simulink model "PMSM"  (R2022a)
settings: Solver=ode23t  StartTime=0.0  StopTime=11  MaxStep=1e-6  RelTol=1e-3
values from neighbouring files (symbols this model uses):
  eps_startup = f/t_startup    (= 40.8333333333)    [PMSM.m]
  J = 0.00000600    (= 6e-06)    [PMSM.m]
  Ls = 0.0002700    (= 0.00027)    [PMSM.m]
  psi = 0.0043319    [PMSM.m]
  Rs = 0.600    (= 0.6)    [PMSM.m]
  t_startup = 10    [PMSM.m]
  zp = 7    [PMSM.m]
libraries: fl_lib x11, nesl_utility x10, ee_lib x1
settings Model: Creator=63250  LastModifiedBy=81502

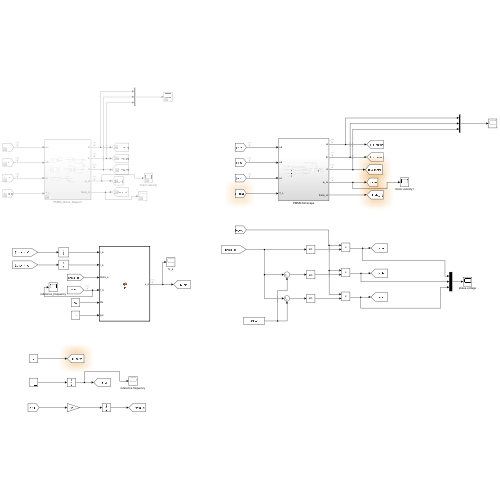
[thumbnail: Simulink's stored preview of the top-level diagram]
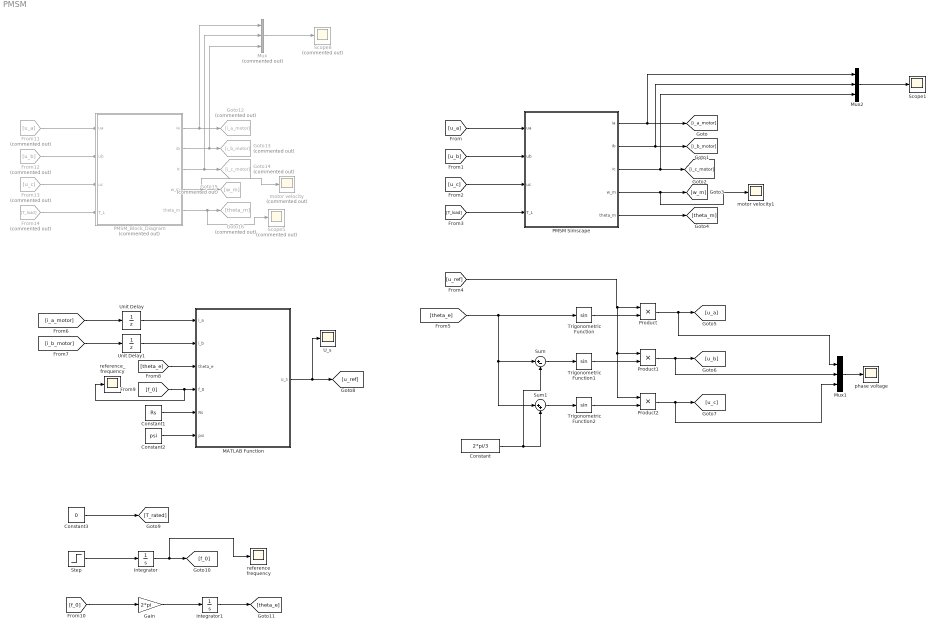
== system PMSM ==
  Constant : Constant  Value=2*pi/3
  Constant1 : Constant  Value=Rs
  Constant2 : Constant  Value=psi
  Constant3 : Constant  Value=0
  From11 : From  Commented=on  GotoTag=u_a
  From12 : From  Commented=on  GotoTag=u_b
  From13 : From  Commented=on  GotoTag=u_c
  From14 : From  Commented=on  GotoTag=T_load
  Gain : Gain  Gain=2*pi
  Goto12 : Goto  Commented=on  GotoTag=i_a_motor
  Goto13 : Goto  Commented=on  GotoTag=i_b_motor
  Goto14 : Goto  Commented=on  GotoTag=i_c_motor
  Goto15 : Goto  Commented=on  GotoTag=w_m
  Goto16 : Goto  Commented=on  GotoTag=theta_m
  Integrator : Integrator
  Integrator1 : Integrator
  MATLAB Function : MATLAB Function  TreatAsAtomicUnit=on
  Mux : Mux  Commented=on  Inputs=3
  Mux1 : Mux  Inputs=3
  Mux2 : Mux  Inputs=3
  PMSM Simscape : Subsystem
  PMSM_Block_Diagram : Subsystem  Commented=on
  Product : Product
  Product1 : Product
  Product2 : Product
  Scope1 : Scope
  Scope5 : Scope  Commented=on
  Scope8 : Scope  Commented=on
  Step : Step  Time=t_startup  Before=eps_startup  After=0  OutDataTypeStr=Inherit: Inherit via back propagation  SampleTime=0
  Sum : Sum  Inputs=|+-
  Sum1 : Sum  Inputs=|++
  Trigonometric Function : Trigonometry
  Trigonometric Function1 : Trigonometry
  Trigonometric Function2 : Trigonometry
  U_s : Scope
  Unit Delay : UnitDelay  SampleTime=-1  HasFrameUpgradeWarning=on
  Unit Delay1 : UnitDelay  SampleTime=-1  HasFrameUpgradeWarning=on
  motor velocity : Scope  Commented=on
  motor velocity1 : Scope
  phase voltage : Scope
  reference frequency : Scope
  reference_frequency : Scope
  wires:
  [u_a] -> PMSM Simscape/1(ua)
  [u_b] -> PMSM Simscape/2(ub)
  [u_c] -> PMSM Simscape/3(uc)
  [T_load] -> PMSM Simscape/4(T_L)
  PMSM Simscape/5(theta_m) -> [theta_m]
  PMSM Simscape/4(w_m) -> motor velocity1/1, [w_m]
  [theta_e] -> Sum/1, Sum1/1, Trigonometric Function/1
  Sum/1 -> Trigonometric Function1/1
  Sum1/1 -> Trigonometric Function2/1
  Constant/1 -> Sum1/2, Sum/2
  Trigonometric Function2/1 -> Product2/2
  Trigonometric Function1/1 -> Product1/2
  Trigonometric Function/1 -> Product/2
  [u_ref] -> Product2/1, Product1/1, Product/1
  [i_a_motor] -> Unit Delay/1
  [i_b_motor] -> Unit Delay1/1
  MATLAB Function/1(u_s) -> U_s/1, [u_ref]
  Unit Delay/1 -> MATLAB Function/1(i_a)
  Unit Delay1/1 -> MATLAB Function/2(i_b)
  [theta_e] -> MATLAB Function/3(theta_e)
  [f_0] -> reference_frequency/1, MATLAB Function/4(f_0)
  Constant1/1 -> MATLAB Function/5(Rs)
  Constant2/1 -> MATLAB Function/6(psi)
  Constant3/1 -> [T_rated]
  Integrator1/1 -> [theta_e]
  Integrator/1 -> reference frequency/1, [f_0]
  Step/1 -> Integrator/1
  [f_0] -> Gain/1
  Gain/1 -> Integrator1/1
  From11/1 -> PMSM_Block_Diagram/1(ua)
  From13/1 -> PMSM_Block_Diagram/3(uc)
  From14/1 -> PMSM_Block_Diagram/4(T_L)
  From12/1 -> PMSM_Block_Diagram/2(ub)
  PMSM_Block_Diagram/2(ib) -> Mux/3, Goto13/1
  PMSM_Block_Diagram/5(theta_m) -> Scope5/1, Goto16/1
  PMSM_Block_Diagram/4(w_m) -> motor velocity/1, Goto15/1
  Mux/1 -> Scope8/1
  PMSM_Block_Diagram/3(ic) -> Goto14/1, Mux/2
  PMSM_Block_Diagram/1(ia) -> Mux/1, Goto12/1
  Mux1/1 -> phase voltage/1
  Product2/1 -> Mux1/3, [u_c]
  Product/1 -> Mux1/1, [u_a]
  Product1/1 -> Mux1/2, [u_b]
  Mux2/1 -> Scope1/1
  PMSM Simscape/1(ia) -> Mux2/1, [i_a_motor]
  PMSM Simscape/3(ic) -> Mux2/3, [i_c_motor]
  PMSM Simscape/2(ib) -> Mux2/2, [i_b_motor]

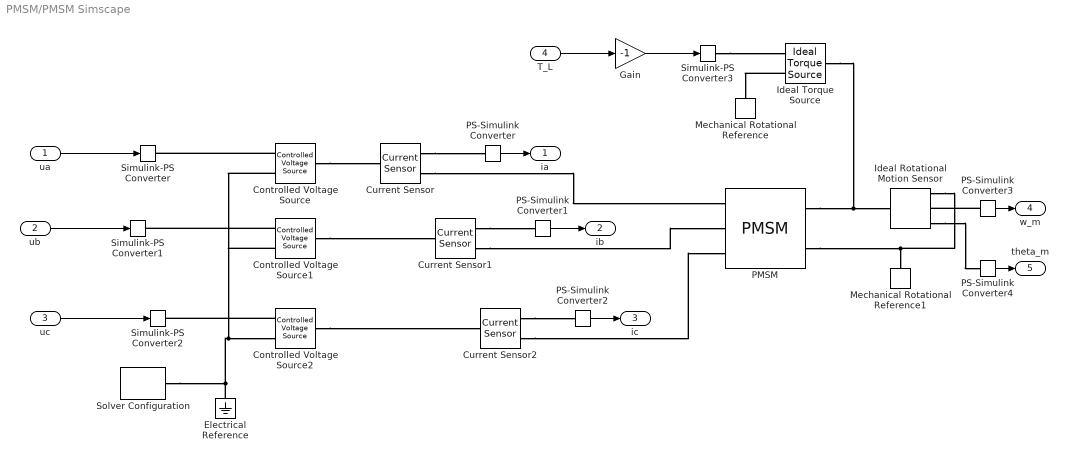
== system PMSM/PMSM Simscape ==
  ua : Inport
  ub : Inport  Port=2
  uc : Inport  Port=3
  T_L : Inport  Port=4
  Controlled Voltage Source : fl_lib/Electrical/Electrical Sources/Controlled Voltage Source
      settings: SourceProductBaseCode=PW,SS,VE
  Controlled Voltage Source1 : fl_lib/Electrical/Electrical Sources/Controlled Voltage Source
      settings: SourceProductBaseCode=PW,SS,VE
  Controlled Voltage Source2 : fl_lib/Electrical/Electrical Sources/Controlled Voltage Source
      settings: SourceProductBaseCode=PW,SS,VE
  Current Sensor : fl_lib/Electrical/Electrical Sensors/Current Sensor
      settings: SourceProductBaseCode=PW,SS,VE
  Current Sensor1 : fl_lib/Electrical/Electrical Sensors/Current Sensor
      settings: SourceProductBaseCode=PW,SS,VE
  Current Sensor2 : fl_lib/Electrical/Electrical Sensors/Current Sensor
      settings: SourceProductBaseCode=PW,SS,VE
  Electrical Reference : fl_lib/Electrical/Electrical Elements/Electrical Reference
      settings: SourceProductBaseCode=PW,SS,VE
  Gain : Gain  Gain=-1
  Ideal Rotational Motion Sensor : fl_lib/Mechanical/Mechanical Sensors/Ideal Rotational Motion Sensor  wrap_angle=simscape.enum.onoff.off  offset=0 rad
      settings: SourceProductBaseCode=PW,SS,VE
  Ideal Torque Source : fl_lib/Mechanical/Mechanical Sources/Ideal Torque Source
      settings: SourceProductBaseCode=PW,SS,VE
  Mechanical Rotational Reference : fl_lib/Mechanical/Rotational Elements/Mechanical Rotational Reference
      settings: SourceProductBaseCode=PW,SS,VE
  Mechanical Rotational Reference1 : fl_lib/Mechanical/Rotational Elements/Mechanical Rotational Reference
      settings: SourceProductBaseCode=PW,SS,VE
  PMSM : ee_lib/Electromechanical/Permanent Magnet/PMSM  port_option=ee.enum.threePhasePort.expanded  winding_type=ee.enum.statorconnection.wye  machine_param=ee.enum.pmsm.parameterization.constant  nPolePairs=zp  pmflux_param=ee.enum.pmflux.fluxlinkage  pm_flux_linkage=psi Wb  torque_constant=0.18 N*m/A  back_emf_constant=0.18 V*s/rad  stator_param=ee.enum.statorparam.LdLqL0  Ld=Ls H  Lq=Ls H  idVec=[-200, 0, 200] A  iqVec=[-200, 0, 200] A  LdMatrix=0.0002 * ones(3, 3) H  LqMatrix=0.0002 * ones(3, 3) H  PmMatrix=0.1 * ones(3, 3) Wb  ktMatrix=0.18 * ones(3, 3) N*m/A  keMatrix=0.18 * ones(3, 3) V*s/rad  L0=Rs H  Ls=0.0002 H  Lm=-0.00002 H  Ms=0.00002 H  Rs=Rs Ohm  zero_sequence=ee.enum.park.zerosequence.exclude  axes_param=ee.enum.rotorangle.daxis  loss_param=ee.enum.ironloss.none  losses_oc=[0, 0, 0] W  losses_sc=[0, 0, 0] W  f_losses=60 Hz  Isc_losses=95 A  J=J kg*m^2  lam=0 N*m*s/rad  i_d_specify=off  i_d_priority=None  i_d=0 A  i_d_nominal_specify=off  i_d_nominal_unit=A  i_d_nominal_value=1  i_q_specify=off  i_q_priority=None  i_q=0 A  i_q_nominal_specify=off  i_q_nominal_unit=A  i_q_nominal_value=1  torque_specify=off  torque_priority=None  torque=0 N*m  torque_nominal_specify=off  torque_nominal_unit=N*m  torque_nominal_value=1  angular_velocity_specify=off  angular_velocity_priority=High  angular_velocity=0 rpm  angular_velocity_nominal_specify=off  angular_velocity_nominal_unit=rpm  angular_velocity_nominal_value=1  angular_position_specify=off  angular_position_priority=High  angular_position=0 deg  angular_position_nominal_specify=off  angular_position_nominal_unit=deg  angular_position_nominal_value=1  alpha=3.93e-3 1/K  alpha_flux=-0.001 1/K  Tmeas=298.15 K  stator_thermal_mass=100 J/K  rotor_thermal_mass=200 J/K  Rm_percent_rotor=90  Rd_percent_rotor=30  temperatureA_specify=off  temperatureA_priority=High  temperatureA=25 degC  temperatureA_nominal_specify=off  temperatureA_nominal_unit=degC  temperatureA_nominal_value=1  temperatureB_specify=off  temperatureB_priority=High  temperatureB=25 degC  temperatureB_nominal_specify=off  temperatureB_nominal_unit=degC  temperatureB_nominal_value=1  temperatureC_specify=off  temperatureC_priority=High  temperatureC=25 degC  temperatureC_nominal_specify=off  temperatureC_nominal_unit=degC  temperatureC_nominal_value=1  temperatureR_specify=off  temperatureR_priority=High  temperatureR=25 degC  temperatureR_nominal_specify=off  temperatureR_nominal_unit=degC  temperatureR_nominal_value=1
      settings: InternalSimscapePortConfiguration="{\"Bottom\":[],\"Left\":[{\"id\":\"a\",\"label\":\"a\",\"type\":\"foundation.electrical.electrical\"},{\"id\":\"b\",\"label\":\"b\",\"type\":\"foundation.electrical.electrical\"},{\"id\":\"c\",\"label\":\"c\",\"type\":\"foundation.electrical.electrical\"}],\"Right\":[{\"id\":\"R\",\"label\":\"R\",\"type\":\"foundation.mechanical.rotational.rotational\"},{\"id\":\"C\",\"label\":\"C\",\"type\":\"foundation.mechanical.rotational.rotational\"}],\"Top\":[]}"
  PS-Simulink Converter{,1..4} (5 alike) : nesl_utility/PS-Simulink Converter  PhysicalDomain=network_engine_domain  SubClassName=ps_output  LeftPortType=input  RightPortType=output  PseudoPeriodic=off  Frequencies=[]  VectorFormat=inherit  Unit=inherit  AffineConversion=off
      settings: SourceProductBaseCode=SS,PW,VE
  Simulink-PS Converter{,1..3} (4 alike) : nesl_utility/Simulink-PS Converter  PhysicalDomain=network_engine_domain  SubClassName=ps_input  LeftPortType=input  RightPortType=output  PseudoPeriodic=off  Frequencies=[]  NoiseDistribution=none  NoiseParameters=[]  Unit=1  AffineConversion=off  FilteringAndDerivatives=provide  SimscapeFilterOrder=1  InputFilterTimeConstant=0.001  UdotUserProvided=0
      settings: SourceProductBaseCode=SS,PW,VE
  Solver Configuration : nesl_utility/Solver Configuration  PhysicalDomain=network_engine_domain  SubClassName=solver  LeftPortType=input  RightPortType=generic  Tones=[]  Harmonics=[]  SimulateNoise=off  Profile=off  UseLocalSampling=off  EnableSwitchedLinearOptims=on  FrequencyDomain=off  UseCCode=off  RelTol=0.001  AbsTol=0.001  MinStep=1e-09  ToWorkspace=off  RevertToSquareIcSolve=off  NumHomotopyIterations=100  PhasorMode=off  PhasorModeNumHarmonics=1  IndexReductionMethod=DerivativeReplacement  DoDC=off  ResidualTolerance=1e-09  UseLocalSolver=off  LocalSolverChoice=NE_BACKWARD_EULER_ADVANCER  LocalSolverSampleTime=0.001  DoFixedCost=off  MaxNonlinIter=3  MaxModeIter=2  ComputeImpulses=off  ImpulseIterations=2  LinearAlgebra=auto  LinearAlgebraNumThread=0  EquationFormulation=NE_TIME_EF  DelaysMemoryBudget=1024  AutomaticFiltering=on  FilteringTimeConstant=0.001  PartitionStorageMethod=AS_NEEDED  PartitionMemoryBudget=1024  PartitionMethod=ROBUST
      settings: SourceProductBaseCode=SS,PW,VE
  ia : Outport
  ib : Outport  Port=2
  ic : Outport  Port=3
  w_m : Outport  Port=4
  theta_m : Outport  Port=5
  wires:
  ua/1 -> Simulink-PS Converter/1
  ub/1 -> Simulink-PS Converter1/1
  uc/1 -> Simulink-PS Converter2/1
  PS-Simulink Converter/1 -> ia/1
  PS-Simulink Converter1/1 -> ib/1
  PS-Simulink Converter2/1 -> ic/1
  T_L/1 -> Gain/1
  Gain/1 -> Simulink-PS Converter3/1
  PS-Simulink Converter3/1 -> w_m/1
  PS-Simulink Converter4/1 -> theta_m/1
  connections:
  Controlled Voltage Source2/RConn1 -- Simulink-PS Converter2/RConn1
  Controlled Voltage Source1/RConn1 -- Simulink-PS Converter1/RConn1
  Controlled Voltage Source/RConn1 -- Simulink-PS Converter/RConn1
  Solver Configuration/RConn1 -- Controlled Voltage Source1/RConn2 -- Controlled Voltage Source/RConn2 -- Controlled Voltage Source2/RConn2 -- Electrical Reference/LConn1
  Controlled Voltage Source/LConn1 -- Current Sensor/LConn1
  Controlled Voltage Source1/LConn1 -- Current Sensor1/LConn1
  Controlled Voltage Source2/LConn1 -- Current Sensor2/LConn1
  Current Sensor/RConn1 -- PS-Simulink Converter/LConn1
  Current Sensor1/RConn1 -- PS-Simulink Converter1/LConn1
  Current Sensor2/RConn1 -- PS-Simulink Converter2/LConn1
  Current Sensor/RConn2 -- PMSM/LConn1
  Current Sensor1/RConn2 -- PMSM/LConn2
  Current Sensor2/RConn2 -- PMSM/LConn3
  Simulink-PS Converter3/RConn1 -- Ideal Torque Source/RConn1
  Ideal Torque Source/RConn2 -- Mechanical Rotational Reference/LConn1
  Ideal Torque Source/LConn1 -- Ideal Rotational Motion Sensor/LConn1 -- PMSM/RConn1
  Ideal Rotational Motion Sensor/RConn1 -- PMSM/RConn2 -- Mechanical Rotational Reference1/LConn1
  PS-Simulink Converter3/LConn1 -- Ideal Rotational Motion Sensor/RConn2
  Ideal Rotational Motion Sensor/RConn3 -- PS-Simulink Converter4/LConn1

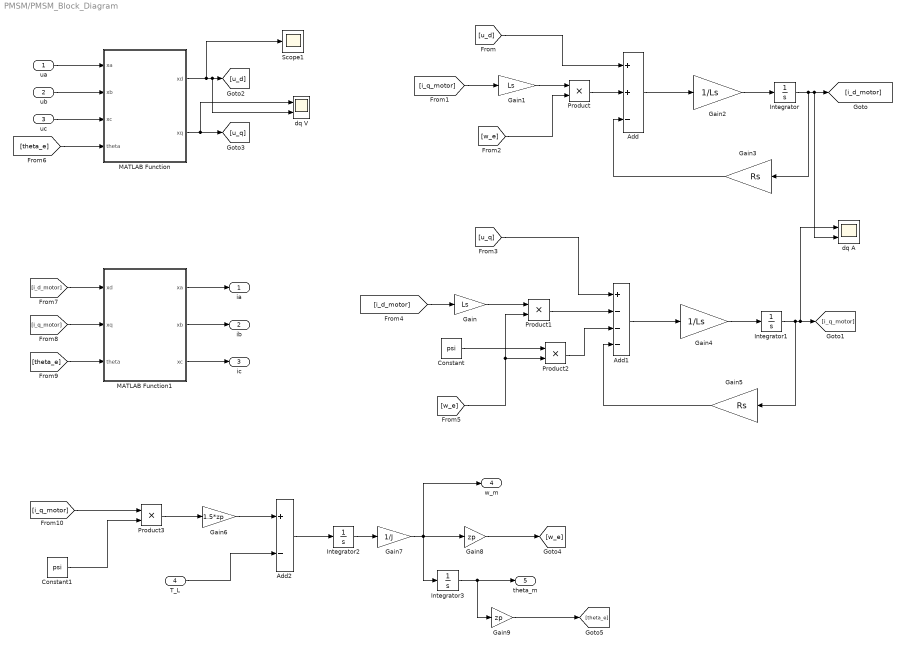
== system PMSM/PMSM_Block_Diagram ==
  ua : Inport
  ub : Inport  Port=2
  uc : Inport  Port=3
  T_L : Inport  Port=4
  Add : Sum  Inputs=++-
  Add1 : Sum  Inputs=+---
  Add2 : Sum  Inputs=+-
  Constant : Constant  Value=psi
  Constant1 : Constant  Value=psi
  Gain : Gain  Gain=Ls
  Gain1 : Gain  Gain=Ls
  Gain2 : Gain  Gain=1/Ls
  Gain3 : Gain  Gain=Rs
  Gain4 : Gain  Gain=1/Ls
  Gain5 : Gain  Gain=Rs
  Gain6 : Gain  Gain=1.5*zp
  Gain7 : Gain  Gain=1/J
  Gain8 : Gain  Gain=zp
  Gain9 : Gain  Gain=zp
  Integrator{,1..3} (4 alike) : Integrator
  MATLAB Function : MATLAB Function  TreatAsAtomicUnit=on
  MATLAB Function1 : MATLAB Function  TreatAsAtomicUnit=on
  Product{,1..3} (4 alike) : Product
  Scope1 : Scope
  dq A : Scope  NumInputPorts=2
  dq V : Scope  NumInputPorts=2
  ia : Outport
  ib : Outport  Port=2
  ic : Outport  Port=3
  w_m : Outport  Port=4
  theta_m : Outport  Port=5
  wires:
  [u_d] -> Add/1
  Product/1 -> Add/2
  [i_q_motor] -> Gain1/1
  Gain1/1 -> Product/1
  [w_e] -> Product/2
  Gain2/1 -> Integrator/1
  Integrator/1 -> Gain3/1, dq A/2, [i_d_motor]
  Add/1 -> Gain2/1
  Gain3/1 -> Add/3
  Gain4/1 -> Integrator1/1
  Integrator1/1 -> Gain5/1, dq A/1, [i_q_motor]
  Add1/1 -> Gain4/1
  Gain5/1 -> Add1/4
  [u_q] -> Add1/1
  Product1/1 -> Add1/2
  Product2/1 -> Add1/3
  Constant/1 -> Product2/1
  [w_e] -> Product1/2, Product2/2
  Gain/1 -> Product1/1
  [i_d_motor] -> Gain/1
  ua/1 -> MATLAB Function/1(xa)
  ub/1 -> MATLAB Function/2(xb)
  [theta_e] -> MATLAB Function/4(theta)
  uc/1 -> MATLAB Function/3(xc)
  MATLAB Function/1(xd) -> Scope1/1, dq V/2, [u_d]
  MATLAB Function/2(xq) -> dq V/1, [u_q]
  [i_d_motor] -> MATLAB Function1/1(xd)
  [i_q_motor] -> MATLAB Function1/2(xq)
  [theta_e] -> MATLAB Function1/3(theta)
  MATLAB Function1/1(xa) -> ia/1
  MATLAB Function1/2(xb) -> ib/1
  MATLAB Function1/3(xc) -> ic/1
  [i_q_motor] -> Product3/1
  Constant1/1 -> Product3/2
  Product3/1 -> Gain6/1
  Gain6/1 -> Add2/1
  T_L/1 -> Add2/2
  Add2/1 -> Integrator2/1
  Integrator2/1 -> Gain7/1
  Gain7/1 -> w_m/1, Integrator3/1, Gain8/1
  Integrator3/1 -> Gain9/1, theta_m/1
  Gain8/1 -> [w_e]
  Gain9/1 -> [theta_e]

== matlab function PMSM/PMSM_Block_Diagram/MATLAB Function ==
  data: xa input; xd output; xb input; xc input; theta input; xq output
function [xd, xq] = abc2dq(xa, xb, xc, theta) 
    sin_t = sin(theta); 
    cos_t = cos(theta); 
    x2 = [2/3 -(1/3) -(1/3); 0 1/sqrt(3) -1/sqrt(3)] * [xa xb xc]';
    x_alpha = x2(1);
    x_beta = x2(2); 
    xd = x_alpha * cos_t + x_beta * sin_t; 
    xq = -x_alpha * sin_t + x_beta * cos_t;
end

== matlab function PMSM/MATLAB Function ==
  data: i_a input; u_s output; i_b input; theta_e input; f_0 input; Rs input; psi input
function  u_s = fcn(i_a, i_b, theta_e, f_0, Rs, psi)
i_s_cos = 2 / 3 * (i_a * cos(theta_e) + i_b * cos(theta_e - 2 * pi /3) - (i_a + i_b) * cos(theta_e + 2 * pi / 3));
i_s = sqrt(1 / 3 * (i_a + 2 * i_b)^2 + i_a^2);
u_s = Rs * i_s_cos + sqrt((2 * pi * f_0 *psi)^2 + (Rs * i_s_cos)^2 - (Rs * i_s)^2);
end

== matlab function PMSM/PMSM_Block_Diagram/MATLAB Function1 ==
  data: xd input; xa output; xq input; theta input; xb output; xc output
function [xa, xb, xc] = dq2abc(xd, xq, theta) 
    sin_t = sin(theta); 
    cos_t = cos(theta); 
    x_alpha = xd * cos_t - xq * sin_t;
    x_beta = xd * sin_t + xq * cos_t; 
    xa = x_alpha;
    xb = (-0.5) * x_alpha + sqrt(3) / 2 * x_beta; 
    xc = (-0.5) * x_alpha - sqrt(3) / 2 * x_beta; 
end
